simulink model "Controller"  (R2019b)
settings: Solver=VariableStepAuto  StartTime=0.0  StopTime=155  RelTol=1e-3
undefined symbols (not defined in the file or in its folder): magnitude
settings Model: Creator=Alex  LastModifiedBy=Alex

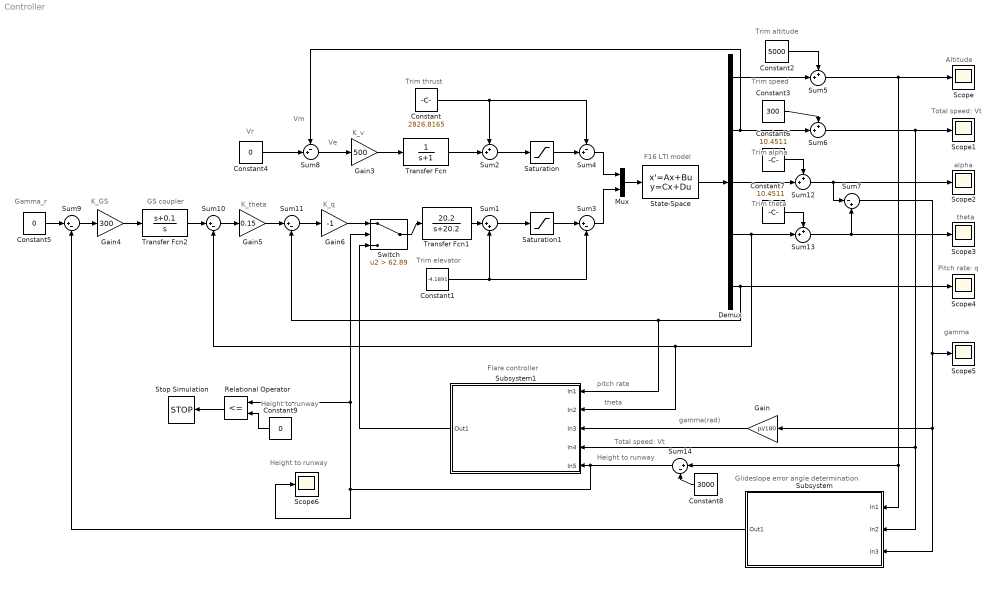
== system Controller ==
  note: Altitude
  note: Total speed: Vt
  note: alpha
  note: theta
  note: Pitch rate: q
  note: Glideslope error angle determination
  note: Trim altitude
  note: Trim speed
  note: Trim thrust
  note: Vr
  note: Vm
  note: Ve
  note: Trim elevator
  note: Gamma_r
  note: K_GS
  note: GS coupler
  note: K_theta
  note: K_q
  note: K_v
  note: Trim alpha
  note: Trim theta
  note: Height to runway
  note: Total speed: Vt
  note: gamma(rad)
  note: pitch rate
  note: theta
  note: gamma
  note: Height to runway
  note: Height to runway
  note: Flare controller
  note: F16 LTI model
  Constant : Constant  Value=2826.8165
  Constant1 : Constant  Value=-4.1891
  Constant2 : Constant  Value=5000
  Constant3 : Constant  Value=300
  Constant4 : Constant  Value=0
  Constant5 : Constant  Value=0
  Constant6 : Constant  Value=10.4511
  Constant7 : Constant  Value=10.4511
  Constant8 : Constant  Value=3000
  Constant9 : Constant  Value=0
  Demux : Demux  Outputs=5
  Gain : Gain  Gain=pi/180
  Gain3 : Gain  Gain=500
  Gain4 : Gain  Gain=300
  Gain5 : Gain  Gain=0.15
  Gain6 : Gain  Gain=-1
  Mux : Mux  Inputs=2
  Relational Operator : RelationalOperator  Operator=<=  OutDataTypeStr=boolean  RndMeth=Simplest
  Saturation : Saturate  UpperLimit=19000  LowerLimit=1000
  Saturation1 : Saturate  UpperLimit=25  LowerLimit=-25
  Scope{,1..6} (7 alike) : Scope
  State-Space : StateSpace  A="[0 0 -300 300 0 ;0.000131652  -0.029096 2.129953 -32.16999 -2.89516 ; 3.15369e-06 -0.0006969  -0.544660 4.5498e-13 0.91522 ;0 0 0 0 1;0 0 0.3303 0 -0.8169 ]"  B=[0 0;0.0015439 -0.004533;-9.493088e-07 -0.0011163;0 0;0 -0.05701634]  C=[1 0 0 0 0;0 1 0 0 0;0 0 180/pi 0 0; 0 0 0 180/pi 0; 0 0 0 0 180/pi]  D=[0 0;0 0;0 0;0 0;0 0]  InitialCondition=[0;0;0;0;0]
  Stop Simulation : Stop
  Subsystem : Subsystem
  Subsystem1 : Subsystem
  Sum1 : Sum  Inputs=|++
  Sum{3,9..11,14} (5 alike) : Sum  Inputs=|+-
  Sum{2,5..6,12..13} (5 alike) : Sum  Inputs=++|
  Sum4 : Sum  Inputs=-+|
  Sum7 : Sum  Inputs=|-+
  Sum8 : Sum  Inputs=-+|
  Switch : Switch  Criteria=u2 > Threshold  Threshold=62.89
  Transfer Fcn : TransferFcn  Denominator=[1 1]
  Transfer Fcn1 : TransferFcn  Numerator=[20.2]  Denominator=[1 20.2]
  Transfer Fcn2 : TransferFcn  Numerator=[1 0.1]  Denominator=[1 0]
  wires:
  Mux/1 -> State-Space/1
  Sum4/1 -> Mux/1
  Saturation/1 -> Sum4/2
  Sum2/1 -> Saturation/1
  Transfer Fcn/1 -> Sum2/2
  Saturation1/1 -> Sum3/1
  Sum1/1 -> Saturation1/1
  Constant/1 -> Sum4/1, Sum2/1
  Constant1/1 -> Sum3/2, Sum1/2
  Demux/1 -> Sum5/2
  Constant2/1 -> Sum5/1
  Sum5/1 -> Scope/1, Subsystem/1(In1), Sum14/1
  Demux/2 -> Sum8/1, Sum6/2
  Constant3/1 -> Sum6/1
  Sum6/1 -> Scope1/1, Subsystem/2(In2), Subsystem1/4(In4)
  Sum7/1 -> Scope5/1, Subsystem/3(In3), Gain/1
  Gain3/1 -> Transfer Fcn/1
  Sum8/1 -> Gain3/1
  Constant4/1 -> Sum8/2
  Constant5/1 -> Sum9/1
  Demux/5 -> Sum11/2, Subsystem1/1(In1), Scope4/1
  Sum9/1 -> Gain4/1
  Gain4/1 -> Transfer Fcn2/1
  Transfer Fcn2/1 -> Sum10/1
  Sum10/1 -> Gain5/1
  Gain5/1 -> Sum11/1
  Sum11/1 -> Gain6/1
  Transfer Fcn1/1 -> Sum1/1
  Subsystem/1(Out1) -> Sum9/2
  Sum3/1 -> Mux/2
  Constant6/1 -> Sum12/1
  Demux/3 -> Sum12/2
  Sum12/1 -> Sum7/1, Scope2/1
  Constant7/1 -> Sum13/1
  Demux/4 -> Sum10/2, Subsystem1/2(In2), Sum13/2
  Sum13/1 -> Sum7/2, Scope3/1
  State-Space/1 -> Demux/1
  Constant8/1 -> Sum14/2
  Sum14/1 -> Scope6/1, Relational Operator/1, Switch/2, Subsystem1/5(In5)
  Switch/1 -> Transfer Fcn1/1
  Gain6/1 -> Switch/1
  Subsystem1/1(Out1) -> Switch/3
  Gain/1 -> Subsystem1/3(In3)
  Constant9/1 -> Relational Operator/2
  Relational Operator/1 -> Stop Simulation/1

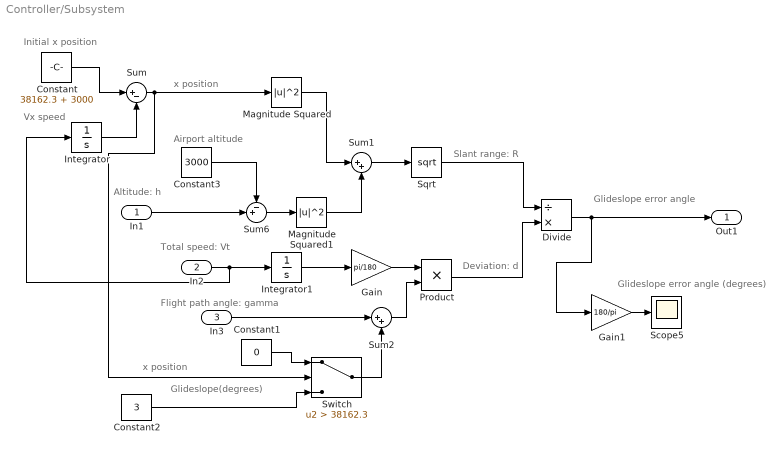
== system Controller/Subsystem ==
  note: Initial x position
  note: Altitude: h
  note: Vx speed
  note: x position
  note: Total speed: Vt
  note: Flight path angle: gamma
  note: Slant range: R
  note: Deviation: d
  note: Glideslope error angle
  note: Airport altitude
  note: Glideslope(degrees)
  note: x position
  note: Glideslope error angle (degrees)
  In1 : Inport
  In2 : Inport  Port=2
  In3 : Inport  Port=3
  Constant : Constant  Value=38162.3 + 3000
  Constant1 : Constant  Value=0
  Constant2 : Constant  Value=3
  Constant3 : Constant  Value=3000
  Divide : Product  Inputs=/*
  Gain : Gain  Gain=pi/180
  Gain1 : Gain  Gain=180/pi
  Integrator : Integrator
  Integrator1 : Integrator
  Magnitude Squared : Math  Operator=magnitude^2  SignedPower=off  SaturateOnIntegerOverflow=on
  Magnitude Squared1 : Math  Operator=magnitude^2  SignedPower=off  SaturateOnIntegerOverflow=on
  Product : Product
  Scope5 : Scope
  Sqrt : Sqrt  SaturateOnIntegerOverflow=on
  Sum : Sum  Inputs=|+-
  Sum1 : Sum  Inputs=|++
  Sum2 : Sum  Inputs=|++
  Sum6 : Sum  Inputs=-+|
  Switch : Switch  Criteria=u2 > Threshold  Threshold=38162.3
  Out1 : Outport
  wires:
  In2/1 -> Integrator/1, Integrator1/1
  Constant/1 -> Sum/1
  Integrator/1 -> Sum/2
  Sum/1 -> Magnitude Squared/1, Switch/2
  Magnitude Squared/1 -> Sum1/1
  Magnitude Squared1/1 -> Sum1/2
  Sum1/1 -> Sqrt/1
  Integrator1/1 -> Gain/1
  Sum2/1 -> Product/2
  Gain/1 -> Product/1
  Sqrt/1 -> Divide/1
  Product/1 -> Divide/2
  In1/1 -> Sum6/2
  Constant3/1 -> Sum6/1
  Sum6/1 -> Magnitude Squared1/1
  In3/1 -> Sum2/1
  Switch/1 -> Sum2/2
  Constant1/1 -> Switch/1
  Constant2/1 -> Switch/3
  Gain1/1 -> Scope5/1
  Divide/1 -> Gain1/1, Out1/1

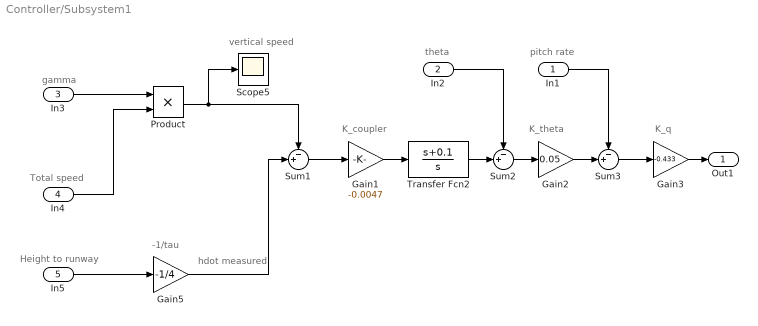
== system Controller/Subsystem1 ==
  note: pitch rate
  note: Total speed
  note: gamma
  note: Height to runway
  note: -1/tau
  note: hdot measured
  note: vertical speed
  note: K_coupler
  note: theta
  note: K_theta
  note: K_q
  In1 : Inport
  In2 : Inport  Port=2
  In3 : Inport  Port=3
  In4 : Inport  Port=4
  In5 : Inport  Port=5
  Gain1 : Gain  Gain=-0.0047
  Gain2 : Gain  Gain=0.05
  Gain3 : Gain  Gain=-0.433
  Gain5 : Gain  Gain=-1/4
  Product : Product
  Scope5 : Scope
  Sum1 : Sum  Inputs=-+|
  Sum2 : Sum  Inputs=-+|
  Sum3 : Sum  Inputs=-+|
  Transfer Fcn2 : TransferFcn  Numerator=[1 0.1]  Denominator=[1 0]
  Out1 : Outport
  wires:
  In4/1 -> Product/2
  In5/1 -> Gain5/1
  Gain5/1 -> Sum1/2
  Product/1 -> Scope5/1, Sum1/1
  Gain1/1 -> Transfer Fcn2/1
  Sum1/1 -> Gain1/1
  Transfer Fcn2/1 -> Sum2/2
  Sum2/1 -> Gain2/1
  Gain2/1 -> Sum3/2
  Sum3/1 -> Gain3/1
  In3/1 -> Product/1
  In2/1 -> Sum2/1
  In1/1 -> Sum3/1
  Gain3/1 -> Out1/1
